simulink model "my_second_model"  (Simulink 8.0)
settings: Solver=ode45  SolverMode=SingleTasking  StartTime=0.0  StopTime=10.0  RelTol=1e-3
libraries: simulink x1
settings Model: Creator=Pranshu  LastModifiedBy=Pranshu  CovMetricSettings=dwe  CovHtmlReporting=off  covSaveCumulativeToWorkspaceVar=off  CovSaveSingleToWorkspaceVar=off  CovExternalEMLEnable=on
settings DataIOCC: LimitDataPoints=off  SaveFormat=StructureWithTime  ReturnWorkspaceOutputs=on
settings OptimizationCC: ExpressionDepthLimit=128
settings DebuggingCC: UnderspecifiedInitializationDetection=Simplified  MergeDetectMultiDrivingBlocksExec=error  SolverPrmCheckMsg=none  FrameProcessingCompatibilityMsg=error  StateNameClashWarn=none  SFUnexpectedBacktrackingDiag=error  SFNoUnconditionalDefaultTransitionDiag=error
settings HardwareCC: ProdBitPerPointer=64  ProdLargestAtomicFloat=Float  ProdIntDivRoundTo=Zero  ProdEndianess=LittleEndian  ProdHWDeviceType=Specified
settings ModelReferenceCC: PropagateSignalLabelsOutOfModel=on
settings SFSimCC: SimUseLocalCustomCode=on
settings RTWCC: RTWUseLocalCustomCode=on
settings CodeAppCC: CustomSymbolStrType=$N$R$M_T
settings GRTTargetCC: CodeReplacementLibrary=C99 (ISO)  GeneratePreprocessorConditionals=Use local settings

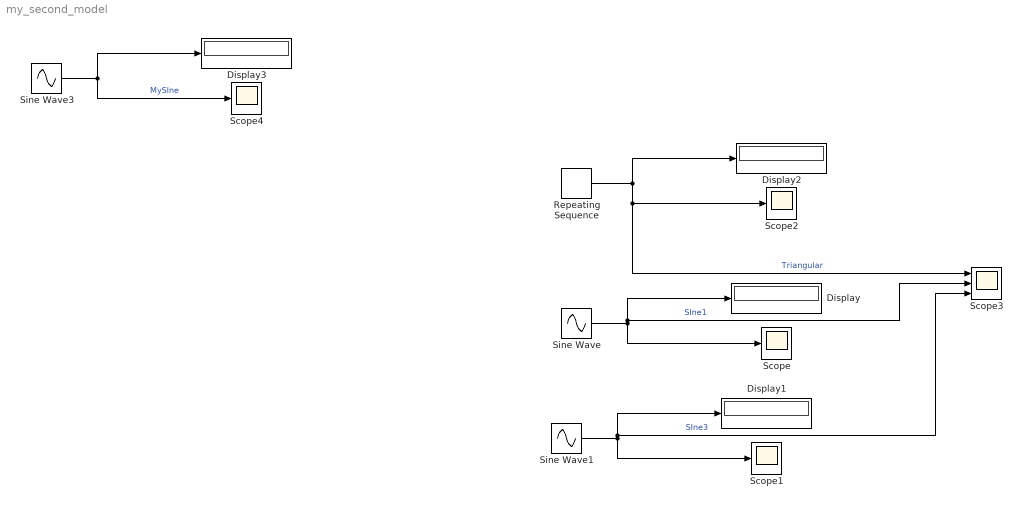
== system my_second_model ==
  Display{,1..3} (4 alike) : Display
  Repeating Sequence : simulink/Sources/Repeating Sequence  rep_seq_t=[0 2]  rep_seq_y=[0 2]
  Scope{,1..2,4} (4 alike) : Scope
      Scope settings: TimeRange=auto  ShowLegends=on  MaxDataPoints=5000  SaveToWorkspace=off  SaveName=ScopeData  YMin=-3.74993  YMax=3.7497  SampleTime=-1
      Scope1 settings: TimeRange=auto  MaxDataPoints=5000  SaveToWorkspace=off  YMin=-1.24563  YMax=1.24904  SampleTime=-1
      Scope2 settings: TimeRange=auto  ShowLegends=on  MaxDataPoints=5000  SaveToWorkspace=off  SaveName=ScopeData2  YMin=-3.73938  YMax=3.7474  SampleTime=-1
      Scope4 settings: TimeRange=auto  ShowLegends=on  MaxDataPoints=5000  SaveToWorkspace=off  YMin=-3.74993  YMax=3.7497  SampleTime=-1
  Scope3 : Scope  NumInputPorts=3
      settings: TimeRange=auto  ShowLegends=on  MaxDataPoints=5000  SaveToWorkspace=off  SaveName=ScopeData3  YMin=-3.74993~-5~-5  YMax=3.7497~5~5  SampleTime=-1
  Sine Wave : Sin  Amplitude=3  Frequency=5  SampleTime=0
  Sine Wave1 : Sin  SampleTime=0
  Sine Wave3 : Sin  Amplitude=3  Frequency=5  SampleTime=0
  wires:
  Sine Wave/1 -> Scope3/2, Display/1, Scope/1  "SIne1"
  Sine Wave1/1 -> Scope3/3, Display1/1, Scope1/1  "SIne3"
  Repeating Sequence/1 -> Display2/1, Scope3/1, Scope2/1  "Triangular"
  Sine Wave3/1 -> Display3/1, Scope4/1  "MySIne"
